simulink model "simulink_model"  (R2022a)
settings: Solver=VariableStepAuto  StartTime=0.0  StopTime=10.0  RelTol=1e-3
libraries: visionsinks x4, sim3dcameralib x1, uavsim3dlib x1, sim3dlib x1, simulink x1
settings Model: Creator=The MathWorks, Inc.  LastModifiedBy=Lenovo
settings SolverCC: AlgebraicLoopSolver=TrustRegion
settings OptimizationCC: ZeroExternalMemoryAtStartup=off  ZeroInternalMemoryAtStartup=off
settings DebuggingCC: UnconnectedInputMsg=warning  UnconnectedOutputMsg=warning  UnconnectedLineMsg=warning
settings SFSimCC: SimTargetLang=C++
settings RTWCC: RTWUseSimCustomCode=on  Toolchain=Simulink Real-Time Remote Build Toolchain  TargetLang=C++  DLArmComputeVersion=19.05
settings CodeAppCC: SimulinkBlockComments=off  MATLABSourceComments=on
settings GRTTargetCC: TargetLangStandard=C++11 (ISO)  CodeInterfacePackaging=C++ class

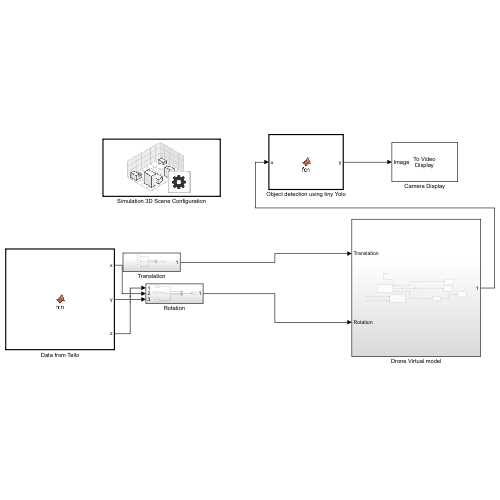
[thumbnail: Simulink's stored preview of the top-level diagram]
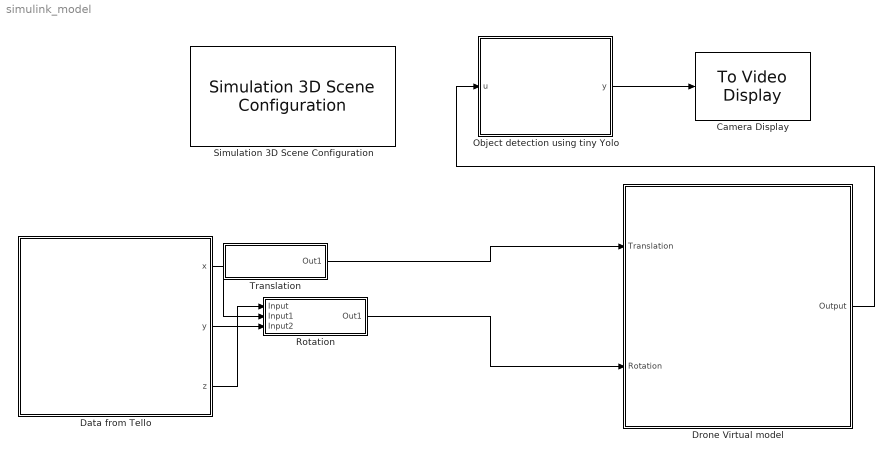
== system simulink_model ==
  Camera Display : visionsinks/To Video Display  windowSizeMode=Normal  openAtMdlStart=on  fullScreen=off  videoWindowX=481  videoWindowY=181  saveWindowSize=off  videoWindowWidth=1280  videoWindowHeight=720  inputColorFormat=RGB  inputType=Obsolete  imagePorts=One multidimensional signal  OutputDevice=On-screen video monitor  dataOrg=Column-major  isWindowOpen=off
  Data from Tello : MATLAB Function  TreatAsAtomicUnit=on
  Drone Virtual model : Subsystem
  Object detection using tiny Yolo : MATLAB Function  TreatAsAtomicUnit=on
  Rotation : Subsystem
  Simulation 3D Scene Configuration : sim3dlib/Simulation 3D Scene Configuration  Priority=0  ProjectFormat=Default Scenes  SceneDesc=US city block  ProjectName=C:\Program Files\MATLAB\R2022a\toolbox\shared\sim3d_projects\automotive_project\UE4\WindowsNoEditor\VehicleSimulation.exe  ScenePath=/Game/Maps/USCityBlock  UEProjPath=D:\Tools2\AutoVrtlEnv\AutoVrtlEnv.uproject  vehTagList={'Scene Origin';'SimulinkVehicle1'}  vehTag=SimulinkVehicle1  OpVisEn=off  Ts=1/60  EnableWindow=on  EnableRemoteAccess=off  EnableWeather=off  SunAltitude=40.0  SunAzimuth=90  clouds=10  wind=1  fog=0  rain=0  sensorTag=MainCamera1  sensorId=1  sensorName=MainCamera1  mountLoc=Origin  offsetFlag=off  tmountOffset=[0, 0, 0]  rmountOffset=[0, 0, 0]  HorizontalResolution=1280  VerticalResolution=720  HorizontalFOV=60  mountPoint=[0 0 0]  mountOrientation=[0 0 0]  aMode=4  ID=1
      settings: SourceProductBaseCode=VE,AE,DR,UV,VE
  Translation : Subsystem
  wires:
  Translation/1(Out1) -> Drone Virtual model/1(Translation)
  Rotation/1(Out1) -> Drone Virtual model/2(Rotation)
  Data from Tello/3(z) -> Rotation/1(Input)
  Data from Tello/2(y) -> Rotation/3(Input2)
  Data from Tello/1(x) -> Rotation/2(Input1)
  Object detection using tiny Yolo/1(y) -> Camera Display/1
  Drone Virtual model/1(Output) -> Object detection using tiny Yolo/1(u)

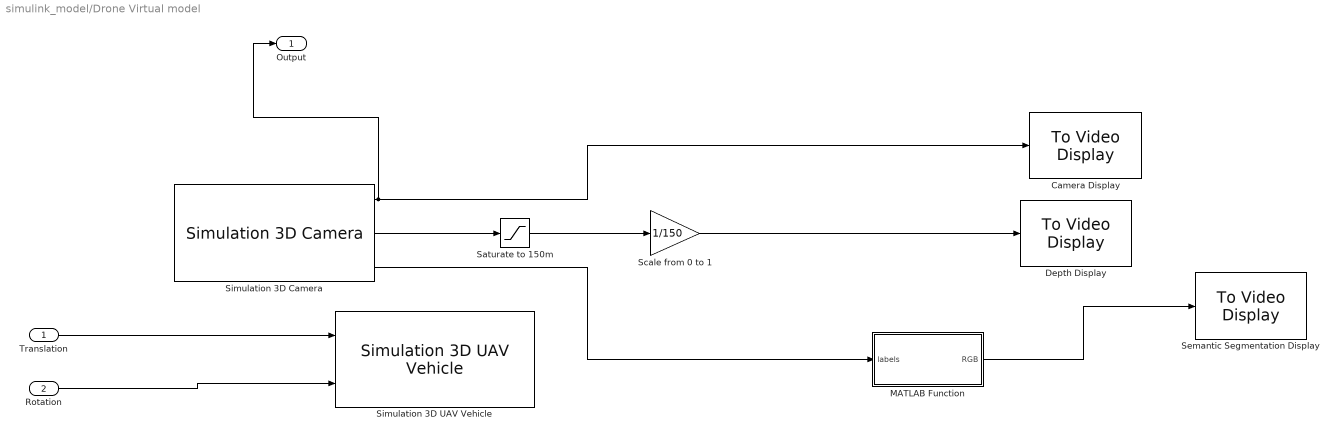
== system simulink_model/Drone Virtual model ==
  Translation : Inport
  Rotation : Inport  Port=2
  Camera Display : visionsinks/To Video Display  windowSizeMode=Normal  openAtMdlStart=on  fullScreen=off  videoWindowX=481  videoWindowY=181  saveWindowSize=off  videoWindowWidth=1280  videoWindowHeight=720  inputColorFormat=RGB  inputType=Obsolete  imagePorts=One multidimensional signal  OutputDevice=On-screen video monitor  dataOrg=Column-major  isWindowOpen=off
  Depth Display : visionsinks/To Video Display  windowSizeMode=Normal  openAtMdlStart=on  fullScreen=off  videoWindowX=497  videoWindowY=162  saveWindowSize=off  videoWindowWidth=1280  videoWindowHeight=720  inputColorFormat=RGB  inputType=Obsolete  imagePorts=One multidimensional signal  OutputDevice=On-screen video monitor  dataOrg=Column-major  isWindowOpen=off
  MATLAB Function : MATLAB Function  TreatAsAtomicUnit=on
  Saturate to 150m : Saturate  UpperLimit=150  LowerLimit=0
  Scale from 0 to 1 : Gain  Gain=1/150
  Semantic Segmentation Display : visionsinks/To Video Display  windowSizeMode=Normal  openAtMdlStart=on  fullScreen=off  videoWindowX=538  videoWindowY=136  saveWindowSize=off  videoWindowWidth=1280  videoWindowHeight=720  inputColorFormat=RGB  inputType=Obsolete  imagePorts=One multidimensional signal  OutputDevice=On-screen video monitor  dataOrg=Column-major  isWindowOpen=off
  Simulation 3D Camera : sim3dcameralib/Simulation 3D Camera  Priority=1  sensorTag=Sim3dSensor1  sensorId=1  sensorName=Sim3dSensor1  vehTagList={'Scene Origin';'SimulinkVehicle1'}  vehTag=SimulinkVehicle1  mountLoc=Origin  offsetFlag=on  tmountOffset=[0.2, 0, 0]  extTmount=off  rmountOffset=[0, 0, 0]  extRmount=off  FocalLength=[1109, 1109]  OpticalCenter=[640, 360]  ImageSize=[720, 1280]  RadialDistortion=[0, 0]  TangentialDistortion=[0, 0]  SensorSkew=0  DepthOutportEnabled=on  SemanticOutportEnabled=on  TransformOutportEnabled=off  SampleTime=-1  mountPoint=[0.2 0 0]  mountOrientation=[0 0 0]  aMode=4  ID=1
      settings: SourceProductBaseCode=VE,AE,DR,UV,VE
  Simulation 3D UAV Vehicle : uavsim3dlib/Simulation 3D UAV Vehicle  Priority=-1  Mesh=Quadrotor  MeshPath=/MathWorksUAVContent/UAVs/HexaRotorUAV/HexaRotor.HexaRotor  Color=Black  ActorName=SimulinkVehicle1  InitialTranslation=[0 0 10]  InitialRotation=[0 0 0]  SampleTime=-1  ActorType=SimulinkVehicle  ID=1  aMode=4  ActorTag=SimulinkVehicle1
      settings: SourceProductBaseCode=UV
  Output : Outport
  wires:
  Simulation 3D Camera/3 -> MATLAB Function/1(labels)
  Scale from 0 to 1/1 -> Depth Display/1
  Saturate to 150m/1 -> Scale from 0 to 1/1
  Simulation 3D Camera/2 -> Saturate to 150m/1
  Translation/1 -> Simulation 3D UAV Vehicle/1
  Rotation/1 -> Simulation 3D UAV Vehicle/2
  Simulation 3D Camera/1 -> Output/1, Camera Display/1
  MATLAB Function/1(RGB) -> Semantic Segmentation Display/1

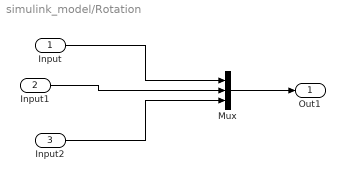
== system simulink_model/Rotation ==
  Input : Inport
  Input1 : Inport  Port=2
  Input2 : Inport  Port=3
  Mux : Mux  Inputs=3
  Out1 : Outport
  wires:
  Mux/1 -> Out1/1
  Input2/1 -> Mux/3
  Input/1 -> Mux/1
  Input1/1 -> Mux/2

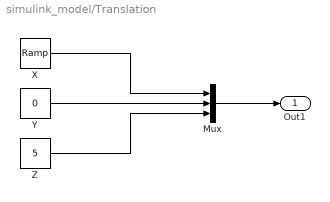
== system simulink_model/Translation ==
  Mux : Mux  Inputs=3
  X : simulink/Sources/Ramp  slope=2  start=0  InitialOutput=0
  Y : Constant  Value=0
  Z : Constant  Value=5
  Out1 : Outport
  wires:
  Mux/1 -> Out1/1
  Z/1 -> Mux/3
  Y/1 -> Mux/2
  X/1 -> Mux/1

== matlab function simulink_model/Data from Tello ==
  data: x output; y output; z output
function [x,y,z]= fcn()
% Create a |ryze| object.
%
% ryzeObj = ryze();
% cameraObj = camera(ryzeObj);
% %  
% serverList = opcuaserverinfo('opc.tcp://LAPTOP-3JNI0QV6:53530/OPCUA/SimulationServer')
% sampleServerInfo = findDescription(serverList, 'Simulation')
% uaClient = opcua('localhost', 53530);
% uaClient = opcua(sampleServerInfo)
% status = uaClient.Status
% 
% isConnected(uaClient)
% % Once you connect the client to the server, additional properties from the server are displayed.
% connect(uaClient)
% uaClient
% uaClient = opcua('localhost', 53530);
% connect(uaClient);

initialValue = 0;  % Initialize with a value that is not possible for 'value'

while true
    tempVariable = findNodeByName(uaClient.Namespace, 'Request', '-once');
    [value, timestamp, quality] = readValue(uaClient, tempVariable);
    tempVariable1 = findNodeByName(uaClient.Namespace, 'Hx', '-once');
    tempVariable2 = findNodeByName(uaClient.Namespace, 'Hy', '-once');
    tempVariable3 = findNodeByName(uaClient.Namespace, 'Hz', '-once');
    
    % Check if the value has changed
    if value ~= initialValue
        % Reset the flag when the value changes
        initialValue = value;

        % Execute the corresponding block
        if value == 1
            takeoff(ryzeObj);
        elseif value == 5
            turn(ryzeObj, deg2rad(90));
            
        elseif value == 2
            video = preview(cameraObj);
            name = "tiny-yolov4-coco";
            detector = yolov4ObjectDetector(name);
            var=1;
            while var<=120
                frame = snapshot(cameraObj);
                [bboxes,scores,labels] = detect(detector, frame);
                detectedFrame = insertObjectAnnotation(frame, 'rectangle', bboxes, labels);
                imshow(detectedFrame);
                var=var+1;
            end
        elseif value == 3
            open('trackBall.m')
            tim = tic;
            duration = 60;
            minGreenIntensity = 40;
            minOffset = 30;
            while toc(tim) < duration
                img = snapshot(cameraObj);
                trackBall(ryzeObj, img, minGreenIntensity, minOffset);
                pause(0.1);
            end
        elseif value == 4
            f = figure;
            hx = animatedline('Color', 'r', 'LineWidth', 2);
            hy = animatedline('Color', 'g', 'LineWidth', 2);
            hz = animatedline('Color', 'b', 'LineWidth', 2);
            title('DroneOrientation v/s Time');
            xlabel('Time (in s)');
            ylabel('Orientation (in degrees)');
            legend('XOrientation', 'YOrientation', 'ZOrientation');
            orientationData = cell(1, 3);
            edgeIndex = 1;
            distance = 5;
            speed = 0.25;
            tObj = tic;
            while edgeIndex <= 4
                % Move the drone unblocking the command line
                tplot = tic;
                moveforward(ryzeObj, 'Distance', distance, 'Speed', speed, 'WaitUntilDone', false);
                % Plot orientation while drone is moving
                while toc(tplot) < distance/speed
                    orientation = rad2deg(readOrientation(ryzeObj));
                                writeValue(uaClient, tempVariable1, orientation(2));
            writeValue(uaClient, tempVariable2, orientation(3));
            writeValue(uaClient, tempVariable3, orientation(1));
                    tStamp = toc(tObj);
                    addpoints(hx, tStamp, orientation(2));
                    addpoints(hy, tStamp, orientation(3));
                    addpoints(hz, tStamp, orientation(1));
                    drawnow;
                    x=orientation(2);
                    y=orientation(3);
                    z=orientation(1);
                    orientationData{end + 1, 1} = tStamp;
        orientationData{end, 2} = orientation(2);
        orientationData{end, 3} = orientation(3);
        orientationData{end, 4} = orientation(1);
                end
                edgeIndex = edgeIndex + 1;
            end
            save('orientation_data.mat', 'orientationData');
        elseif value == 6
            moveforward(ryzeObj, 'Distance', 5, 'Speed', 0.5, 'WaitUntilDone', false);
        end
    end
end

== matlab function simulink_model/Drone Virtual model/MATLAB Function ==
  data: labels input; RGB output
function RGB = uavlabel2rgb(labels)
% Convert semantic segmentation map captured during 3D simulation to RGB
% color image.

% Declare label2rgb function.
coder.extrinsic('label2rgb');

% Preallocate memory for RGB matrix.
RGB = coder.nullcopy(zeros(size(labels,1),size(labels,2),3,class(labels)));

% Define colormap using 3D simulation label IDs.
cmap = sim3dColormap;

% Convert labels to RGB color image.
RGB = label2rgb(labels, cmap);

== matlab function simulink_model/Object detection using tiny Yolo ==
  data: u input; y output
function y = fcn(u)

y = u;
